simulink model "txline_filter_rab"  (Simulink 7.4)
settings: Solver=ode45  StartTime=0.0  StopTime=10  RelTol=1e-3
undefined symbols (not defined in the file or in its folder): Fs, magnitude
libraries: rftxlines1 x6, dspindex x6, rfports1 x4, dspsigops x3, dspsnks4 x2, dspbuff3 x2, dspxfrm3 x2, dsparch3 x2, simulink x1, dspmtrx3 x1, dspsrcs4 x1
settings Model: Creator=RobertZ  LastModifiedBy=Dick
settings DataIOCC: SaveOutput=off  SaveTime=off  SignalLoggingName=sigsOut
settings OptimizationCC: InlineInvariantSignals=on  InitFltsAndDblsToZero=on
settings DebuggingCC: SaveWithParameterizedLinksMsg=none  CheckExecutionContextPreStartOutputMsg=on  CheckExecutionContextRuntimeOutputMsg=on  SignalResolutionControl=TryResolveAllWithWarning  SolverPrmCheckMsg=none  MultiTaskDSMMsg=warning  MultiTaskCondExecSysMsg=none  StrictBusMsg=None
settings HardwareCC: ProdHWDeviceType=Specified
settings ModelReferenceCC: UpdateModelReferenceTargets=IfOutOfDate
settings RTWCC: IncludeERTFirstTime=on
settings GRTTargetCC: TargetFcnLib=ansi_tfl_tmw.mat

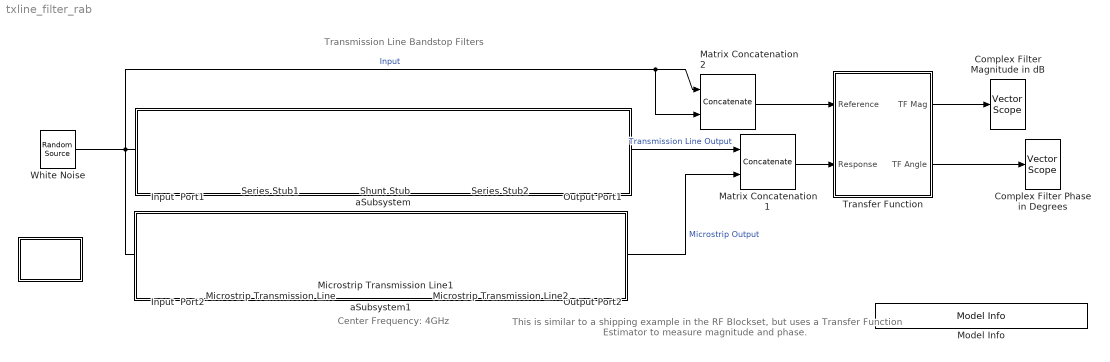
== system txline_filter_rab ==
  note: Transmission Line Bandstop Filters
  note: Center Frequency: 4GHz
  note: This is similar to a shipping example in the RF Blockset, but uses a
      | Transfer Function Estimator to measure magnitude and phase.
  " " : Subsystem
      mask Type: Interpolation filter info block
      mask Display: disp('Info')
  Complex Filter Magnitude in dB : dspsnks4/Vector Scope  DialogController=dspdialog.VectorScope  DialogControllerArgs=DataTag0  ScopeProperties=on  Domain=Frequency  HorizSpan=1  DisplayProperties=off  AxisGrid=on  Memory=off  FrameNumber=on  AxisLegend=off  AxisZoom=off  OpenScopeAtSimStart=on  OpenScopeImmediately=off  FigPos=[75 330 372 236]  AxisProperties=off  XUnits=Hertz  XRange=[-Fs/2...Fs/2]  InheritXIncr=on  XIncr=2*Fs  XLabel=Time  XLimit=Auto  XMin=0  XMax=1  XStart=0  YUnits=dB  YLabel=dB  LineProperties=off  LineColors=[0 1 1]|[1 0 0]  XAxisParamsVer=6.8
      settings: YMin=-29.6158045438743  YMax=-6.27914514640088
  Complex Filter Phase in Degrees : dspsnks4/Vector Scope  DialogController=dspdialog.VectorScope  DialogControllerArgs=DataTag1  ScopeProperties=on  Domain=Frequency  HorizSpan=1  DisplayProperties=off  AxisGrid=on  Memory=off  FrameNumber=on  AxisLegend=off  AxisZoom=off  OpenScopeAtSimStart=on  OpenScopeImmediately=off  FigPos=[457 331 372 236]  AxisProperties=off  XUnits=Hertz  XRange=[-Fs/2...Fs/2]  InheritXIncr=on  XIncr=1  XLabel=Frequency  XLimit=Auto  XMin=0  XMax=1  XStart=0  YUnits=Magnitude  YLabel=Phase in Degrees  LineProperties=off  LineColors=[0 1 1]|[1 0 0]  XAxisParamsVer=6.8
      settings: YMin=-351.310972463598  YMax=440.341024264227
  Input  Port1 : rfports1/Input Port  Description=source block  DialogController=rfblksDDGCreate  DialogControllerArgs=DataTag2  SystemSampleTime=-1  TreatSimulinkInputSignalAs=Source voltage  MaxLength=160  FracBW=0  ModelDelay=0  Fc=4e9  Ts=1/5e9  Zs=50  NoiseFlag=off  seed=67987  GoToTag=BAEFFHHQSZBERFFHEUVSUCG
  Input  Port2 : rfports1/Input Port  Description=source block  DialogController=rfblksDDGCreate  DialogControllerArgs=DataTag3  SystemSampleTime=-1  TreatSimulinkInputSignalAs=Source voltage  MaxLength=160  FracBW=0  ModelDelay=0  Fc=4e9  Ts=1/5e9  Zs=50  NoiseFlag=off  seed=67987  GoToTag=BAEACLDICAAIGSJKBYZDYGF
  Matrix Concatenation1 : Concatenate  Mode=Multidimensional array  ConcatenateDimension=2
  Matrix Concatenation2 : Concatenate  Mode=Multidimensional array  ConcatenateDimension=2
  Microstrip Transmission Line : rftxlines1/Microstrip Transmission Line  DialogController=rfblksDDGCreate  DialogControllerArgs=DataTag4  PhysicalDomain=rfsystemsdomain  SubClassName=microstrip  LeftPortType=p1  RightPortType=p1  LConnTagsString=__newl0  RConnTagsString=__newr0  Width=2.6501e-3  Height=0.635e-3  Thickness=0.01e-3  EpsilonR=9.8  LossTangent=0  SigmaCond=inf  LineLength=0.00663  StubMode=Series  Termination=Short  PlotFreq=Derived from Input Port parameters  SourceFreq=User-specified  Freq=1.5e9:10e6:6.5e9  AllPlotType=X-Y plane  AppliedNetworkData=S21  AppliedComplexFormat=Angle (degrees)  AppliedNetworkData2=""  AppliedXParameter=Freq  AppliedXFormat=Hz  YOption=Linear  XOption=Linear  PlotZ0=50  DisplayData=off  PlotFreqNoSim=User-specified  NetworkData=S21  SmithData=S11  PolarData=S11  ComplexFormat=Magnitude (decibels)  DBFormat=Magnitude (decibels)  NoneFormat=None
  Microstrip Transmission Line1 : rftxlines1/Microstrip Transmission Line  DialogController=rfblksDDGCreate  DialogControllerArgs=DataTag5  PhysicalDomain=rfsystemsdomain  SubClassName=microstrip  LeftPortType=p1  RightPortType=p1  LConnTagsString=__newl0  RConnTagsString=__newr0  Width=0.40564e-3  Height=0.635e-3  Thickness=0.01e-3  EpsilonR=9.8  LossTangent=0  SigmaCond=inf  LineLength=0.00735  StubMode=Shunt  Termination=Open  PlotFreq=Derived from Input Port parameters  SourceFreq=User-specified  Freq=1.5e9:10e6:6.5e9  AllPlotType=X-Y plane  AppliedNetworkData=S21  AppliedComplexFormat=Angle (degrees)  AppliedNetworkData2=""  AppliedXParameter=Freq  AppliedXFormat=Hz  YOption=Linear  XOption=Linear  PlotZ0=50  DisplayData=off  PlotFreqNoSim=User-specified  NetworkData=S21  SmithData=S11  PolarData=S11  ComplexFormat=Magnitude (decibels)  DBFormat=Magnitude (decibels)  NoneFormat=None
  Microstrip Transmission Line2 : rftxlines1/Microstrip Transmission Line  DialogController=rfblksDDGCreate  DialogControllerArgs=DataTag6  PhysicalDomain=rfsystemsdomain  SubClassName=microstrip  LeftPortType=p1  RightPortType=p1  LConnTagsString=__newl0  RConnTagsString=__newr0  Width=2.6501e-3  Height=0.635e-3  Thickness=0.01e-3  EpsilonR=9.8  LossTangent=0  SigmaCond=inf  LineLength=0.00663  StubMode=Series  Termination=Short  PlotFreq=Derived from Input Port parameters  SourceFreq=User-specified  Freq=1.5e9:10e6:6.5e9  AllPlotType=X-Y plane  AppliedNetworkData=S21  AppliedComplexFormat=Angle (degrees)  AppliedNetworkData2=""  AppliedXParameter=Freq  AppliedXFormat=Hz  YOption=Linear  XOption=Linear  PlotZ0=50  DisplayData=off  PlotFreqNoSim=User-specified  NetworkData=S21  SmithData=S11  PolarData=S11  ComplexFormat=Magnitude (decibels)  DBFormat=Magnitude (decibels)  NoneFormat=None
  Model Info : simulink/Model-Wide Utilities/Model Info  SystemSampleTime=-1  InitialBlockCM=None  BlockCM=None  Frame=on  DisplayStringWithTags=Copywrite 2005-2010 The MathWorks, Inc.  HorizontalTextAlignment=Center  LeftAlignmentValue=0.5  SourceBlockDiagram=txline_filter_rab  TagMaxNumber=20
  Output Port1 : rfports1/Output Port  DialogController=rfblksDDGCreate  DialogControllerArgs=DataTag7  SystemSampleTime=-1  Zl=50  Flag=0  num_Models=1  GoToTag=BAEFFHHQSZBERFFHEUVSUCG  PlotFreq=Derived from Input Port parameters  SourceFreq=Derived from Input Port parameters  Freq=1e9:1e8:3e9  AllPlotType=Composite data  AppliedNetworkData=S11  AppliedComplexFormat=Magnitude (decibels)  AppliedNetworkData2=""  AppliedXParameter=Freq  AppliedXFormat=Hz  YOption=Linear  XOption=Linear  PlotZ0=50  DisplayData=off  NoBudgetPlot=Composite data  NetworkData=S11  SmithData=S11  PolarData=S11  ComplexFormat=Magnitude (decibels)  DBFormat=Magnitude (decibels)  DBMFormat=dBm  NoneFormat=None
  Output Port2 : rfports1/Output Port  DialogController=rfblksDDGCreate  DialogControllerArgs=DataTag8  SystemSampleTime=-1  Zl=50  Flag=0  num_Models=1  GoToTag=BAEACLDICAAIGSJKBYZDYGF  PlotFreq=Derived from Input Port parameters  SourceFreq=Derived from Input Port parameters  Freq=1e9:1e8:3e9  AllPlotType=Composite data  AppliedNetworkData=S11  AppliedComplexFormat=Magnitude (decibels)  AppliedNetworkData2=""  AppliedXParameter=Freq  AppliedXFormat=Hz  YOption=Linear  XOption=Linear  PlotZ0=50  DisplayData=off  NoBudgetPlot=Composite data  NetworkData=S11  SmithData=S11  PolarData=S11  ComplexFormat=Magnitude (decibels)  DBFormat=Magnitude (decibels)  DBMFormat=dBm  NoneFormat=None
  Series Stub1 : rftxlines1/Transmission Line  DialogController=rfblksDDGCreate  DialogControllerArgs=DataTag9  PhysicalDomain=rfsystemsdomain  SubClassName=txline  LeftPortType=p1  RightPortType=p1  LConnTagsString=__newl0  RConnTagsString=__newr0  Z0=20.71  PV=1.8e8  Loss=0  ParamFreq=1e9  InterpMethod=Linear  LineLength=0.0113  StubMode=Series  Termination=Short  PlotFreq=Derived from Input Port parameters  SourceFreq=User-specified  Freq=1.5e9:10e6:6.5e9  AllPlotType=X-Y plane  AppliedNetworkData=S21  AppliedComplexFormat=Angle (degrees)  AppliedNetworkData2=""  AppliedXParameter=Freq  AppliedXFormat=Hz  YOption=Linear  XOption=Linear  PlotZ0=50  DisplayData=off  PlotFreqNoSim=User-specified  NetworkData=S21  SmithData=S11  PolarData=S11  ComplexFormat=Magnitude (decibels)  DBFormat=Magnitude (decibels)  NoneFormat=None
  Series Stub2 : rftxlines1/Transmission Line  DialogController=rfblksDDGCreate  DialogControllerArgs=DataTag10  PhysicalDomain=rfsystemsdomain  SubClassName=txline  LeftPortType=p1  RightPortType=p1  LConnTagsString=__newl0  RConnTagsString=__newr0  Z0=20.71  PV=1.8e8  Loss=0  ParamFreq=1e9  InterpMethod=Linear  LineLength=0.0113  StubMode=Series  Termination=Short  PlotFreq=Derived from Input Port parameters  SourceFreq=User-specified  Freq=1.5e9:10e6:6.5e9  AllPlotType=X-Y plane  AppliedNetworkData=S21  AppliedComplexFormat=Angle (degrees)  AppliedNetworkData2=""  AppliedXParameter=Freq  AppliedXFormat=Hz  YOption=Linear  XOption=Linear  PlotZ0=50  DisplayData=off  PlotFreqNoSim=User-specified  NetworkData=S21  SmithData=S11  PolarData=S11  ComplexFormat=Magnitude (decibels)  DBFormat=Magnitude (decibels)  NoneFormat=None
  Shunt Stub : rftxlines1/Transmission Line  DialogController=rfblksDDGCreate  DialogControllerArgs=DataTag11  PhysicalDomain=rfsystemsdomain  SubClassName=txline  LeftPortType=p1  RightPortType=p1  LConnTagsString=__newl0  RConnTagsString=__newr0  Z0=60.355  PV=1.8e8  Loss=0  ParamFreq=1e9  InterpMethod=Linear  LineLength=0.0113  StubMode=Shunt  Termination=Open  PlotFreq=Derived from Input Port parameters  SourceFreq=User-specified  Freq=1.5e9:10e6:6.5e9  AllPlotType=X-Y plane  AppliedNetworkData=S21  AppliedComplexFormat=Angle (degrees)  AppliedNetworkData2=""  AppliedXParameter=Freq  AppliedXFormat=Hz  YOption=Linear  XOption=Linear  PlotZ0=50  DisplayData=off  PlotFreqNoSim=User-specified  NetworkData=S21  SmithData=S11  PolarData=S11  ComplexFormat=Magnitude (decibels)  DBFormat=Magnitude (decibels)  NoneFormat=None
  "Transfer Function " : Subsystem  mask{NFFT=1024, Navg=100, pcnt=100/1.28, unwrap_flag=off}
      mask prompts: NFFT "FFT length (power of 2):"; Navg "Spectral Averaging Factor (>=1):"; pcnt "Percentage of  Alias Free Data  (<=100)"; unwrap_flag "Unwrap Phase"
      mask Display: disp('Transfer Function \n Estimation (v2.0) ')
  White Noise : dspsrcs4/Random Source  SrcType=Gaussian  NormMethod=Ziggurat  CltLength=12  MinVal=-1.25  MaxVal=1.25  MeanVal=0  VarVal=1  RepMode=Not repeatable  rawSeed=1  IsInherit=off  SampMode=Discrete  SampTime=1/5e9  SampFrame=256  DataType=Double  OutComplex=Complex
  aSubsystem : Subsystem
      mask Display: disp('')
  aSubsystem1 : Subsystem
      mask Display: disp('')
  wires:
  White Noise/1 -> Input  Port1/1, Input  Port2/1, Matrix Concatenation2/1, Matrix Concatenation2/2  "Input"
  Output Port1/1 -> Matrix Concatenation1/1  "Transmission Line Output"
  Output Port2/1 -> Matrix Concatenation1/2  "Microstrip Output"
  Matrix Concatenation1/1 -> "Transfer Function "/2(Response)
  Matrix Concatenation2/1 -> "Transfer Function "/1(Reference)
  "Transfer Function "/1(TF Mag) -> Complex Filter Magnitude in dB/1
  "Transfer Function "/2(TF Angle) -> Complex Filter Phase in Degrees/1
  connections:
  Series Stub1/LConn1 -- Input  Port1/RConn1
  Series Stub1/RConn1 -- Shunt Stub/LConn1
  Shunt Stub/RConn1 -- Series Stub2/LConn1
  Series Stub2/RConn1 -- Output Port1/LConn1
  Input  Port2/RConn1 -- Microstrip Transmission Line/LConn1
  Microstrip Transmission Line/RConn1 -- Microstrip Transmission Line1/LConn1
  Microstrip Transmission Line1/RConn1 -- Microstrip Transmission Line2/LConn1
  Microstrip Transmission Line2/RConn1 -- Output Port2/LConn1

== system txline_filter_rab/  ==
  note: Transmission Line Bandstop Filters
      |
      | The RF Blockset has the following blocks for transmission lines:
      | Coaxial Transmission Line
      | Transmission Line
      | Microstrip Transmission Line
      | Parallel Plate Transmission Line
      | Two Wire Transmission Line
      | Coplanar Waveguide Transmission Line
      |
      | This demo simulates a bandstop Transmission Line filter and
      | a bandstop Microstrip filter with a Gaussian random signal input.
      |
      | The spectrum plot shows frequency ranging from
      | 1.5GHz to 6.5GHz centered at 4GHz.
      |
      |
      | If you want to see the frequency response centered at other RF frequency,
      | you need to change the Center frequency parameter in the
      | 'Input Port' block.
      |
      | If you want to change the range of frequency response that is determined by
      | the Sample time parameter specified in the 'Input Port' and 'White Noise' blocks,
      | you need to change the Sample time parameter in both blocks.

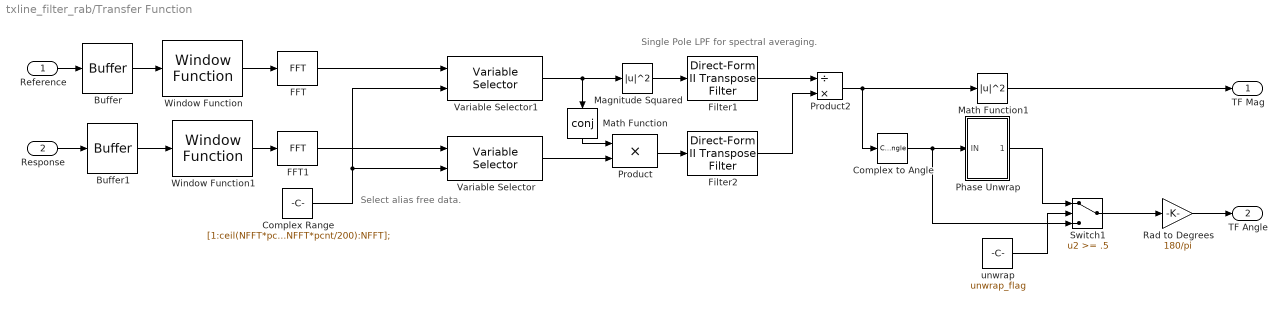
== system txline_filter_rab/Transfer Function  ==
  note: Single Pole LPF for spectral averaging.
  note: Select alias free data.
  Reference : Inport  OutDataType=sfix(16)  OutScaling=2^0
  Response : Inport  Port=2  OutDataType=sfix(16)  OutScaling=2^0
  Buffer : dspbuff3/Buffer  N=NFFT  V=0  ic=0
  Buffer1 : dspbuff3/Buffer  N=NFFT  V=0  ic=0
  Complex Range : Constant  Value=[1:ceil(NFFT*pcnt/200),ceil(1+NFFT-NFFT*pcnt/200):NFFT];  OutDataType=sfix(16)  OutScaling=2^0
  Complex to Angle : ComplexToMagnitudeAngle  Output=Angle
  FFT : dspxfrm3/FFT  DialogController=dspDDGCreate  DialogControllerArgs=DataTag12  CompMethod=Table lookup  TableOpt=HYBRID  TableOptActive=Speed  BitRevOrder=off  InheritFFTLength=on  FFTLength=64  SkipNorm=on  firstCoeffMode=Specify word length  firstCoeffWordLength=16  firstCoeffFracLength=15  roundingMode=Floor  overflowMode=off
  FFT1 : dspxfrm3/FFT  DialogController=dspDDGCreate  DialogControllerArgs=DataTag13  CompMethod=Table lookup  TableOpt=HYBRID  TableOptActive=Speed  BitRevOrder=off  InheritFFTLength=on  FFTLength=64  SkipNorm=on  firstCoeffMode=User-defined  firstCoeffWordLength=16  firstCoeffFracLength=15  roundingMode=Floor  overflowMode=off
  Filter1 : dsparch3/Direct-Form II Transpose Filter  num=1  den=[Navg -(Navg-1)]  ic=eps
  Filter2 : dsparch3/Direct-Form II Transpose Filter  num=1  den=[Navg -(Navg-1)]  ic=eps
  Magnitude Squared : Math  Operator=magnitude^2  OutDataType=sfix(16)  OutScaling=2^0  SaturateOnIntegerOverflow=on
  Math Function : Math  Operator=conj  OutDataType=sfix(16)  OutScaling=2^0  SaturateOnIntegerOverflow=on
  Math Function1 : Math  Operator=magnitude^2  OutDataType=sfix(16)  OutScaling=2^0  SaturateOnIntegerOverflow=on
  Phase Unwrap : Subsystem
  Product : Product  OutDataType=sfix(16)  OutScaling=2^0  SaturateOnIntegerOverflow=on  InputSameDT=on  OutDataTypeStr=Inherit: Same as first input
  Product2 : Product  Inputs=/*  OutDataType=sfix(16)  OutScaling=2^0  SaturateOnIntegerOverflow=on  InputSameDT=on  OutDataTypeStr=Inherit: Same as first input
  Rad to Degrees : Gain  Gain=180/pi  ParameterDataType=sfix(16)  ParameterScaling=2^0  OutDataType=sfix(16)  OutScaling=2^0
  Switch1 : Switch  Threshold=.5
  Variable Selector : dspindex/Variable Selector  NumInputs=1  rowsOrCols=Rows  IdxMode=Variable  Elements=[1 3]  ZerOneIdxMode=One-based  errmode=Clip Index  FillMode=on  FillValues=0
  Variable Selector1 : dspindex/Variable Selector  NumInputs=1  rowsOrCols=Rows  IdxMode=Variable  Elements=[1 3]  ZerOneIdxMode=One-based  errmode=Clip Index  FillMode=on  FillValues=0
  Window Function : dspsigops/Window Function  DialogController=dspDDGCreate  DialogControllerArgs=DataTag15  winmode=Apply window to input  wintype=Hann  sampmode=Continuous  samptime=1  N=64  Rs=50  beta=10  winsamp=Periodic  UserWindow=hamming  OptParams=off  UserParams={'symmetric'}  dataType=double  isSigned=on  wordLen=16  udDataType=sfix(16)  fracBitsMode=Best precision  numFracBits=15  roundingMode=Floor  overflowMode=off  numSidelobes=4  sidelobeLevel=-30
  Window Function1 : dspsigops/Window Function  DialogController=dspDDGCreate  DialogControllerArgs=DataTag16  winmode=Apply window to input  wintype=Hann  sampmode=Continuous  samptime=1  N=64  Rs=50  beta=10  winsamp=Periodic  UserWindow=hamming  OptParams=off  UserParams={'symmetric'}  dataType=double  isSigned=on  wordLen=16  udDataType=sfix(16)  fracBitsMode=Best precision  numFracBits=15  roundingMode=Floor  overflowMode=off  numSidelobes=4  sidelobeLevel=-30
  unwrap : Constant  Value=unwrap_flag  OutDataType=sfix(16)  OutScaling=2^0
  TF Mag : Outport  OutDataType=sfix(16)  OutScaling=2^0
  TF Angle : Outport  Port=2  OutDataType=sfix(16)  OutScaling=2^0
  wires:
  Complex Range/1 -> Variable Selector/2, Variable Selector1/2
  Complex to Angle/1 -> Switch1/3, Phase Unwrap/1(IN)
  Rad to Degrees/1 -> TF Angle/1
  Response/1 -> Buffer1/1
  Reference/1 -> Buffer/1
  Product/1 -> Filter2/1
  FFT1/1 -> Variable Selector/1
  Math Function/1 -> Product/1
  Magnitude Squared/1 -> Filter1/1
  FFT/1 -> Variable Selector1/1
  Math Function1/1 -> TF Mag/1
  Window Function/1 -> FFT/1
  Window Function1/1 -> FFT1/1
  Filter1/1 -> Product2/1
  Filter2/1 -> Product2/2
  Buffer/1 -> Window Function/1
  Buffer1/1 -> Window Function1/1
  Product2/1 -> Complex to Angle/1, Math Function1/1
  Variable Selector/1 -> Product/2
  Variable Selector1/1 -> Magnitude Squared/1, Math Function/1
  Switch1/1 -> Rad to Degrees/1
  unwrap/1 -> Switch1/2
  Phase Unwrap/1(Out1) -> Switch1/1

== system txline_filter_rab/aSubsystem ==

== system txline_filter_rab/aSubsystem1 ==

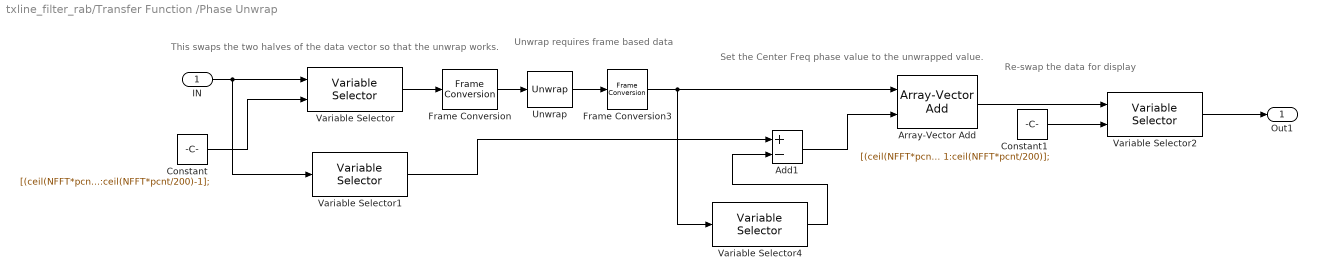
== system txline_filter_rab/Transfer Function /Phase Unwrap ==
  note: This swaps the two halves of the data vector
      | so that the unwrap works.
  note: Set the Center Freq phase value to the unwrapped value.
  note: Re-swap the data for display
  note: Unwrap requires frame based data
  IN : Inport  OutDataType=sfix(16)  OutScaling=2^0
  Add1 : Sum  Inputs=+-  OutDataType=sfix(16)  OutScaling=2^-10
  Array-Vector Add : dspmtrx3/Array-Vector Add  DialogController=dspDDGCreate  DialogControllerArgs=DataTag14  Dimension=2  V_Source=Input port  V_VectFromMask=[0.5 0.25]  firstCoeffDataTypeStr=Inherit: Same word length as input  firstCoeffLastDataTypeStr=Inherit: Same word length as input  firstCoeffMin=[]  firstCoeffMax=[]  outputDataTypeStr=Inherit: Same as accumulator  outputLastDataTypeStr=Inherit: Same as accumulator  outputMin=[]  outputMax=[]  roundingMode=Floor  overflowMode=off
  Constant : Constant  Value=[(ceil(NFFT*pcnt/200)):ceil(NFFT*pcnt/100) 1:ceil(NFFT*pcnt/200)-1];  OutDataType=sfix(16)  OutScaling=2^0
  Constant1 : Constant  Value=[(ceil(NFFT*pcnt/200)+1):ceil(NFFT*pcnt/100) 1:ceil(NFFT*pcnt/200)];  OutDataType=sfix(16)  OutScaling=2^0
  Frame Conversion : FrameConversion
  Frame Conversion3 : FrameConversion  OutFrame=Sample-based
  Unwrap : dspsigops/Unwrap  running=on  tol=pi
  Variable Selector : dspindex/Variable Selector  NumInputs=1  rowsOrCols=Rows  IdxMode=Variable  Elements=[1 3]  ZerOneIdxMode=One-based  errmode=Clip Index  FillMode=on  FillValues=0
  Variable Selector1 : dspindex/Variable Selector  NumInputs=1  rowsOrCols=Rows  IdxMode=Fixed  Elements=[1]  ZerOneIdxMode=One-based  errmode=Clip Index  FillMode=on  FillValues=0
  Variable Selector2 : dspindex/Variable Selector  NumInputs=1  rowsOrCols=Rows  IdxMode=Variable  Elements=[1 3]  ZerOneIdxMode=One-based  errmode=Clip Index  FillMode=on  FillValues=0
  Variable Selector4 : dspindex/Variable Selector  NumInputs=1  rowsOrCols=Rows  IdxMode=Fixed  Elements=length([(ceil(NFFT*pcnt/200)+1):ceil(NFFT*pcnt/100) 1:ceil(NFFT*pcnt/200)] )/2+1  ZerOneIdxMode=One-based  errmode=Clip Index  FillMode=on  FillValues=0
  Out1 : Outport  OutDataType=sfix(16)  OutScaling=2^0
  wires:
  Frame Conversion/1 -> Unwrap/1
  Variable Selector2/1 -> Out1/1
  IN/1 -> Variable Selector/1, Variable Selector1/1
  Constant/1 -> Variable Selector/2
  Variable Selector/1 -> Frame Conversion/1
  Variable Selector1/1 -> Add1/1
  Unwrap/1 -> Frame Conversion3/1
  Variable Selector4/1 -> Add1/2
  Constant1/1 -> Variable Selector2/2
  Frame Conversion3/1 -> Variable Selector4/1, Array-Vector Add/1
  Add1/1 -> Array-Vector Add/2
  Array-Vector Add/1 -> Variable Selector2/1
